simulink model "gyro_processing_test"  (R2016b)
settings: Solver=VariableStepAuto  StartTime=0.0  StopTime=100  RelTol=1e-3
libraries: dynamics_lib x1, sensor_processing_libs x1, gyroscope_lib x1
settings Model: Creator=Sean  LastModifiedBy=taylorreynolds

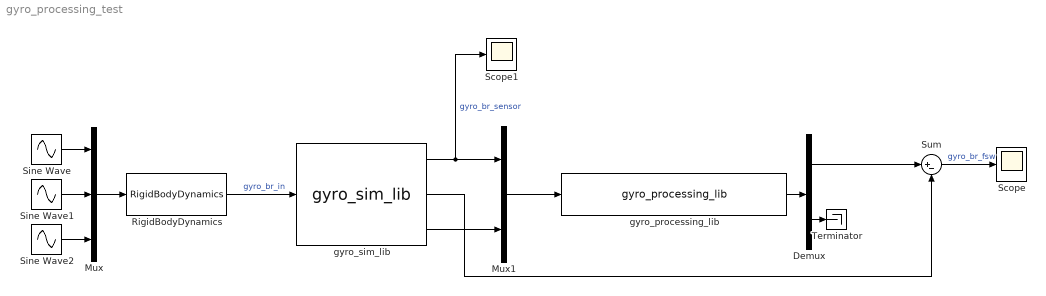
== system gyro_processing_test ==
  Demux : Demux  Outputs=[3 1]
  Mux : Mux  Inputs=3
  Mux1 : Mux  Inputs=[3 1]
  RigidBodyDynamics : dynamics_lib/Dynamics/RigidBodyDynamics
  Scope : Scope
  Scope1 : Scope
  Sine Wave : Sin  Amplitude=2e-4  SampleTime=0
  Sine Wave1 : Sin  Amplitude=2e-4  Phase=pi/3  SampleTime=0
  Sine Wave2 : Sin  Amplitude=2e-4  Phase=2*pi/3  SampleTime=0
  Sum : Sum  Inputs=|+-
  Terminator : Terminator
  gyro_processing_lib : sensor_processing_libs/gyro_processing_lib
  gyro_sim_lib : gyroscope_lib/gyro_sim_lib
  wires:
  RigidBodyDynamics/1 -> gyro_sim_lib/1  "gyro_br_in"
  Mux1/1 -> gyro_processing_lib/1
  gyro_sim_lib/3 -> Mux1/2
  gyro_sim_lib/1 -> Scope1/1, Mux1/1  "gyro_br_sensor"
  Sum/1 -> Scope/1  "gyro_br_fsw"
  gyro_sim_lib/2 -> Sum/2
  gyro_processing_lib/1 -> Demux/1
  Demux/1 -> Sum/1
  Demux/2 -> Terminator/1
  Mux/1 -> RigidBodyDynamics/1
  Sine Wave1/1 -> Mux/2
  Sine Wave/1 -> Mux/1
  Sine Wave2/1 -> Mux/3
